simulink model "single_magnet_single_superconductor"  (R2014a)
settings: Solver=ode45  StartTime=0.0  StopTime=sim_time  RelTol=1e-16
values from neighbouring files (symbols this model uses):
  damping = evalin('base', 'damping')    [FP_sandbox.m]
  mu_FC = [mu_FC_x; mu_FC_y; mu_FC_z]    [FP_sandbox.m]
  mu_mag_0 = evalin('base','mu_mag_0')    [FP_sandbox.m]
  r_FC = [pos_FC_x; pos_FC_y; pos_FC_z]    [FP_sandbox.m]
  r_mag_0 = evalin('base', 'r_mag_0')    [FP_sandbox.m]
undefined symbols (not defined in the file or in its folder): Quat_A0
libraries: simulink x1, vrlib x1
settings Model: Creator=user  LastModifiedBy=user

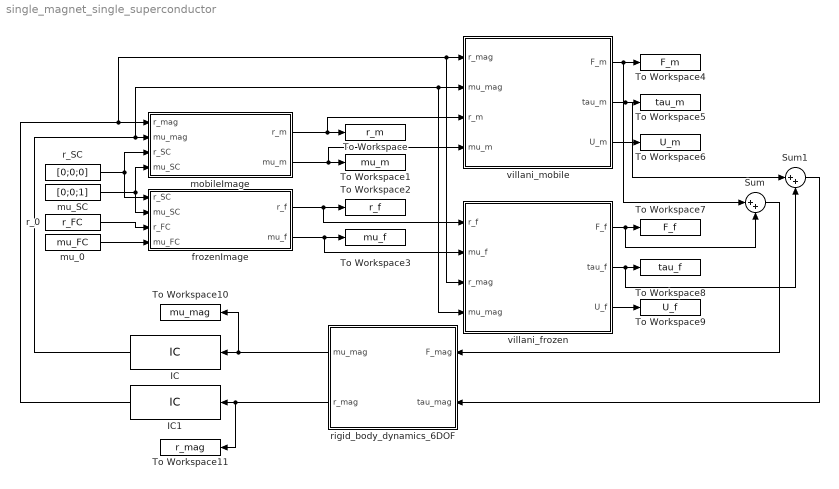
== system single_magnet_single_superconductor ==
  IC : InitialCondition  Value=mu_mag_0
  IC1 : InitialCondition  Value=r_mag_0
  Sum : Sum  Inputs=|++
  Sum1 : Sum  Inputs=|++
  To Workspace : ToWorkspace  VariableName=r_m  SaveFormat=Timeseries  SampleTime=-1
  To Workspace1 : ToWorkspace  VariableName=mu_m  SaveFormat=Timeseries  SampleTime=-1
  To Workspace10 : ToWorkspace  VariableName=mu_mag  SaveFormat=Timeseries  SampleTime=-1
  To Workspace11 : ToWorkspace  VariableName=r_mag  SaveFormat=Timeseries  SampleTime=-1
  To Workspace2 : ToWorkspace  VariableName=r_f  SaveFormat=Timeseries  SampleTime=-1
  To Workspace3 : ToWorkspace  VariableName=mu_f  SaveFormat=Timeseries  SampleTime=-1
  To Workspace4 : ToWorkspace  VariableName=F_m  SaveFormat=Timeseries  SampleTime=-1
  To Workspace5 : ToWorkspace  VariableName=tau_m  SaveFormat=Timeseries  SampleTime=-1
  To Workspace6 : ToWorkspace  VariableName=U_m  SaveFormat=Timeseries  SampleTime=-1
  To Workspace7 : ToWorkspace  VariableName=F_f  SaveFormat=Timeseries  SampleTime=-1
  To Workspace8 : ToWorkspace  VariableName=tau_f  SaveFormat=Timeseries  SampleTime=-1
  To Workspace9 : ToWorkspace  VariableName=U_f  SaveFormat=Timeseries  SampleTime=-1
  frozenImage : MATLAB Function  TreatAsAtomicUnit=on
  mobileImage : MATLAB Function  TreatAsAtomicUnit=on
  mu_0 : Constant  Value=mu_FC
  mu_SC : Constant  Value=[0;0;1]
  r_0 : Constant  Value=r_FC
  r_SC : Constant  Value=[0;0;0]
  "rigid_body_dynamics_6DOF " : Subsystem
  villani_frozen : MATLAB Function  TreatAsAtomicUnit=on
  villani_mobile : MATLAB Function  TreatAsAtomicUnit=on
  wires:
  r_SC/1 -> frozenImage/1(r_SC), mobileImage/3(r_SC)
  mu_SC/1 -> frozenImage/2(mu_SC), mobileImage/4(mu_SC)
  r_0/1 -> frozenImage/3(r_FC)
  mu_0/1 -> frozenImage/4(mu_FC)
  IC/1 -> villani_frozen/4(mu_mag), villani_mobile/2(mu_mag), mobileImage/2(mu_mag)
  IC1/1 -> villani_frozen/3(r_mag), villani_mobile/1(r_mag), mobileImage/1(r_mag)
  mobileImage/1(r_m) -> villani_mobile/3(r_m), To Workspace/1
  mobileImage/2(mu_m) -> villani_mobile/4(mu_m), To Workspace1/1
  frozenImage/1(r_f) -> villani_frozen/1(r_f), To Workspace2/1
  frozenImage/2(mu_f) -> villani_frozen/2(mu_f), To Workspace3/1
  villani_mobile/1(F_m) -> Sum/1, To Workspace4/1
  villani_mobile/2(tau_m) -> Sum1/1, To Workspace5/1
  villani_mobile/3(U_m) -> To Workspace6/1
  villani_frozen/1(F_f) -> Sum/2, To Workspace7/1
  villani_frozen/2(tau_f) -> Sum1/2, To Workspace8/1
  villani_frozen/3(U_f) -> To Workspace9/1
  Sum1/1 -> "rigid_body_dynamics_6DOF "/2(tau_mag)
  Sum/1 -> "rigid_body_dynamics_6DOF "/1(F_mag)
  "rigid_body_dynamics_6DOF "/1(mu_mag) -> To Workspace10/1, IC/1
  "rigid_body_dynamics_6DOF "/2(r_mag) -> To Workspace11/1, IC1/1

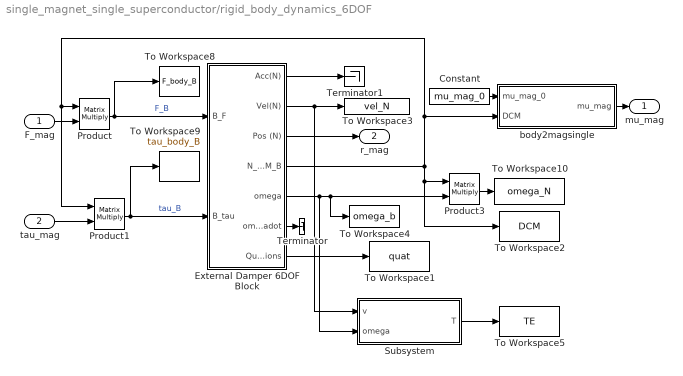
== system single_magnet_single_superconductor/rigid_body_dynamics_6DOF  ==
  F_mag : Inport
  tau_mag : Inport  Port=2
  Constant : Constant  Value=mu_mag_0
  External Damper 6DOF Block : Subsystem  AncestorBlock=OS_Sim_library/External Damper 6DOF block Collision Block
  Product : Product  Multiplication=Matrix(*)
  Product1 : Product  Multiplication=Matrix(*)
  Product3 : Product  Multiplication=Matrix(*)
  Subsystem : Subsystem
  Terminator : Terminator
  Terminator1 : Terminator
  To Workspace1 : ToWorkspace  VariableName=quat  SaveFormat=Timeseries  SampleTime=-1
  To Workspace10 : ToWorkspace  VariableName=omega_N  SaveFormat=Timeseries  SampleTime=-1
  To Workspace2 : ToWorkspace  VariableName=DCM  SaveFormat=Structure With Time  SampleTime=-1
  To Workspace3 : ToWorkspace  VariableName=vel_N  SaveFormat=Timeseries  SampleTime=-1
  To Workspace4 : ToWorkspace  VariableName=omega_b  SaveFormat=Timeseries  SampleTime=-1
  To Workspace5 : ToWorkspace  VariableName=TE  SaveFormat=Timeseries  SampleTime=-1
  To Workspace8 : ToWorkspace  VariableName=F_body_B  SaveFormat=Timeseries  SampleTime=-1
  To Workspace9 : ToWorkspace  VariableName=tau_body_B  SaveFormat=Timeseries  SampleTime=-1
  body2magsingle : MATLAB Function  TreatAsAtomicUnit=on
  mu_mag : Outport
  r_mag : Outport  Port=2
  wires:
  External Damper 6DOF Block/1(Acc(N)) -> Terminator1/1
  External Damper 6DOF Block/6(omegadot) -> Terminator/1
  External Damper 6DOF Block/2(Vel(N)) -> Subsystem/1(v), To Workspace3/1
  body2magsingle/1(mu_mag) -> mu_mag/1
  tau_mag/1 -> Product1/2
  F_mag/1 -> Product/2
  External Damper 6DOF Block/4(N_DCM_B) -> Product1/1, Product/1, body2magsingle/2(DCM), Product3/1, To Workspace2/1
  Product1/1 -> External Damper 6DOF Block/2(B_tau), To Workspace9/1  "tau_B"
  Product/1 -> External Damper 6DOF Block/1(B_F), To Workspace8/1  "F_B"
  External Damper 6DOF Block/3(Pos (N)) -> r_mag/1
  Product3/1 -> To Workspace10/1
  External Damper 6DOF Block/5(omega) -> Product3/2, To Workspace4/1, Subsystem/2(omega)
  External Damper 6DOF Block/7(Quaternions) -> To Workspace1/1
  Subsystem/1(T) -> To Workspace5/1
  Constant/1 -> body2magsingle/1(mu_mag_0)

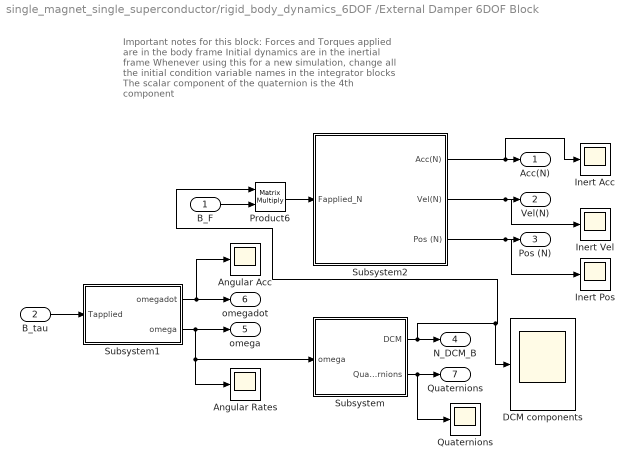
== system single_magnet_single_superconductor/rigid_body_dynamics_6DOF /External Damper 6DOF Block ==
  note: Important notes for this block:
      | Forces and Torques applied are in the body frame
      | Initial dynamics are in the inertial frame
      | Whenever using this for a new simulation, change all the initial condition variable names in the integrator blocks
      | The scalar component of the quaternion is the 4th component
  B_F : Inport
  B_tau : Inport  Port=2
  Angular Acc : Scope
      settings: SaveName=ScopeData30
  Angular Rates : Scope
      settings: SaveName=ScopeData31
  DCM components : Scope
      settings: SaveName=ScopeData34
  Inert Acc : Scope
      settings: SaveName=ScopeData20
  Inert Pos : Scope
      settings: SaveName=ScopeData22
  Inert Vel : Scope
      settings: SaveName=ScopeData21
  Product6 : Product  Multiplication=Matrix(*)  RndMeth=Zero
  "Quaternions " : Scope
      settings: SaveName=ScopeData33
  Subsystem : Subsystem
  Subsystem1 : Subsystem
  Subsystem2 : Subsystem
  Acc(N) : Outport
  Vel(N) : Outport  Port=2  PortDimensions=[3 1]
  Pos (N) : Outport  Port=3
  N_DCM_B : Outport  Port=4
  omega : Outport  Port=5  PortDimensions=[3 1]
  omegadot : Outport  Port=6
  Quaternions : Outport  Port=7
  wires:
  Product6/1 -> Subsystem2/1(Fapplied_N)
  Subsystem/2(Quaternions) -> Quaternions/1, "Quaternions "/1
  Subsystem/1(DCM) -> N_DCM_B/1, Product6/1, DCM components/1
  Subsystem1/1(omegadot) -> omegadot/1, Angular Acc/1
  Subsystem1/2(omega) -> Angular Rates/1, Subsystem/1(omega), omega/1
  B_tau/1 -> Subsystem1/1(Tapplied)
  Subsystem2/1(Acc(N)) -> Inert Acc/1, Acc(N)/1
  Subsystem2/2(Vel(N)) -> Inert Vel/1, Vel(N)/1
  Subsystem2/3(Pos (N)) -> Inert Pos/1, Pos (N)/1
  B_F/1 -> Product6/2

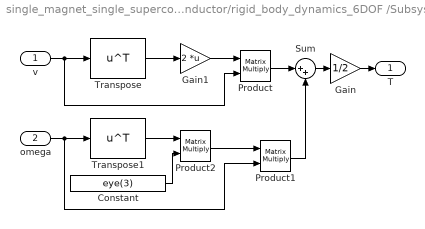
== system single_magnet_single_superconductor/rigid_body_dynamics_6DOF /Subsystem ==
  v : Inport
  omega : Inport  Port=2
  Constant : Constant  Value=eye(3)
  Gain : Gain  Gain=1/2
  Gain1 : Gain  Gain=2  Multiplication=Matrix(K*u)
  Product : Product  Multiplication=Matrix(*)
  Product1 : Product  Multiplication=Matrix(*)
  Product2 : Product  Multiplication=Matrix(*)
  Sum : Sum  Inputs=|++
  Transpose : Math  Operator=transpose  SaturateOnIntegerOverflow=on
  Transpose1 : Math  Operator=transpose  SaturateOnIntegerOverflow=on
  T : Outport  PortDimensions=1
  wires:
  v/1 -> Product/2, Transpose/1
  Transpose/1 -> Gain1/1
  Gain1/1 -> Product/1
  Sum/1 -> Gain/1
  Gain/1 -> T/1
  omega/1 -> Product1/2, Transpose1/1
  Transpose1/1 -> Product2/1
  Product2/1 -> Product1/1
  Product/1 -> Sum/1
  Product1/1 -> Sum/2
  Constant/1 -> Product2/2

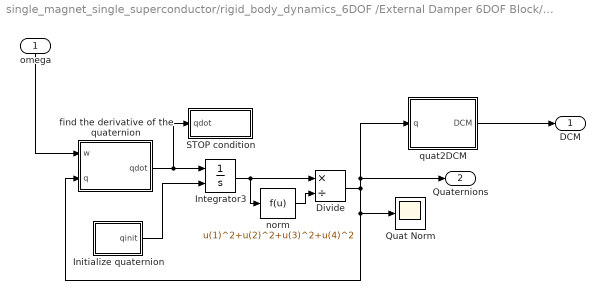
== system single_magnet_single_superconductor/rigid_body_dynamics_6DOF /External Damper 6DOF Block/Subsystem ==
  omega : Inport
  Divide : Product  Inputs=*/
  Initialize quaternion : Subsystem
  Integrator3 : Integrator  InitialConditionSource=external  InitialCondition=Quat_A0
  Quat Norm : Scope
      settings: YMin=-0.1  YMax=1  SaveName=ScopeData32
  STOP condition : Subsystem
  find the derivative of the quaternion : MATLAB Function  TreatAsAtomicUnit=on
  norm : Fcn  Expr=u(1)^2+u(2)^2+u(3)^2+u(4)^2
  quat2DCM : MATLAB Function  TreatAsAtomicUnit=on
  DCM : Outport
  Quaternions : Outport  Port=2
  wires:
  Initialize quaternion/1(qinit) -> Integrator3/2
  quat2DCM/1(DCM) -> DCM/1
  find the derivative of the quaternion/1(qdot) -> STOP condition/1(qdot), Integrator3/1
  Divide/1 -> quat2DCM/1(q), Quaternions/1, find the derivative of the quaternion/2(q), Quat Norm/1
  Integrator3/1 -> Divide/1, norm/1
  omega/1 -> find the derivative of the quaternion/1(w)
  norm/1 -> Divide/2

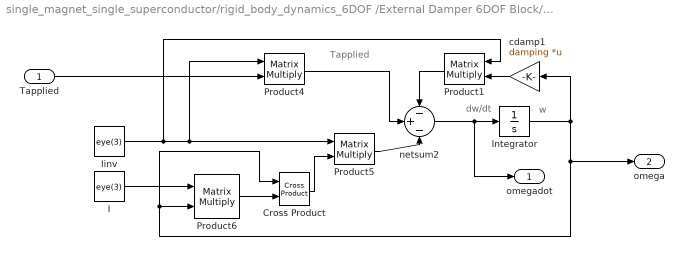
== system single_magnet_single_superconductor/rigid_body_dynamics_6DOF /External Damper 6DOF Block/Subsystem1 ==
  note: dw/dt
  note: w
  note: Tapplied
  Tapplied : Inport
  Cross Product : vrlib/Utilities/Cross Product
  I : Constant  Value=eye(3)  VectorParams1D=off
  Iinv : Constant  Value=eye(3)  VectorParams1D=off
  Integrator : Integrator  InitialCondition=[0 0 0]'
  Product{1,4..6} (4 alike) : Product  Multiplication=Matrix(*)  RndMeth=Zero
  cdamp1 : Gain  Gain=damping  Multiplication=Matrix(K*u)
  netsum2 : Sum  Inputs=-+-  SaturateOnIntegerOverflow=on  InputSameDT=on  OutDataTypeStr=Inherit: Same as first input
  omegadot : Outport
  omega : Outport  Port=2
  wires:
  Cross Product/1 -> Product5/2
  Product4/1 -> netsum2/2
  Product5/1 -> netsum2/3
  Iinv/1 -> Product1/1, Product4/1, Product5/1
  Tapplied/1 -> Product4/2
  Product6/1 -> Cross Product/2
  I/1 -> Product6/1
  netsum2/1 -> Integrator/1, omegadot/1
  Integrator/1 -> omega/1, Cross Product/1, Product6/2, cdamp1/1
  cdamp1/1 -> Product1/2
  Product1/1 -> netsum2/1

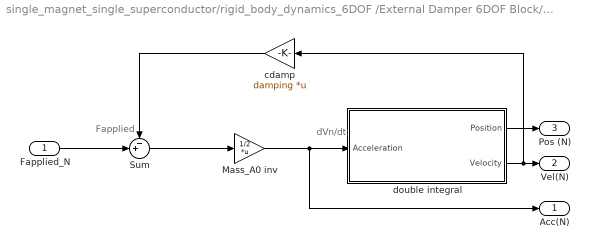
== system single_magnet_single_superconductor/rigid_body_dynamics_6DOF /External Damper 6DOF Block/Subsystem2 ==
  note: dVn/dt
  note: Fapplied
  Fapplied_N : Inport
  Mass_A0 inv : Gain  Gain=1/2  Multiplication=Matrix(K*u)
  Sum : Sum  Inputs=-+|  SaturateOnIntegerOverflow=on
  cdamp : Gain  Gain=damping  Multiplication=Matrix(K*u)
  double integral : Subsystem
  Acc(N) : Outport
  Vel(N) : Outport  Port=2
  Pos (N) : Outport  Port=3
  wires:
  double integral/2(Velocity) -> Vel(N)/1, cdamp/1
  double integral/1(Position) -> Pos (N)/1
  Mass_A0 inv/1 -> double integral/1(Acceleration), Acc(N)/1
  Sum/1 -> Mass_A0 inv/1
  Fapplied_N/1 -> Sum/2
  cdamp/1 -> Sum/1

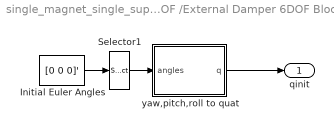
== system single_magnet_single_superconductor/rigid_body_dynamics_6DOF /External Damper 6DOF Block/Subsystem/Initialize quaternion ==
  Initial Euler Angles : Constant  Value=[0 0 0]'
  Selector1 : Selector  InputPortWidth=3  Indices=[3 2 1]
  yaw,pitch,roll to quat : MATLAB Function  TreatAsAtomicUnit=on
  qinit : Outport
  wires:
  yaw,pitch,roll to quat/1(q) -> qinit/1
  Selector1/1 -> yaw,pitch,roll to quat/1(angles)
  Initial Euler Angles/1 -> Selector1/1

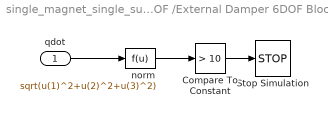
== system single_magnet_single_superconductor/rigid_body_dynamics_6DOF /External Damper 6DOF Block/Subsystem/STOP condition ==
  qdot : Inport
  Compare To Constant : simulink/Logic and Bit Operations/Compare To Constant  relop=>  const=10  OutDataTypeStr=boolean
  Stop Simulation : Stop
  norm : Fcn  Expr=sqrt(u(1)^2+u(2)^2+u(3)^2)
  wires:
  Compare To Constant/1 -> Stop Simulation/1
  norm/1 -> Compare To Constant/1
  qdot/1 -> norm/1

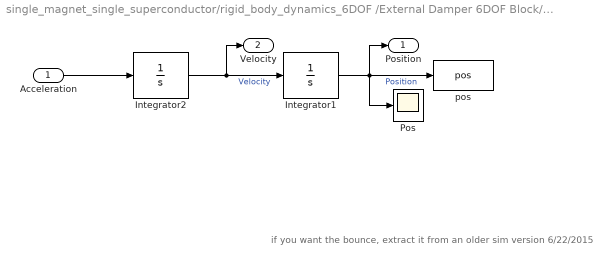
== system single_magnet_single_superconductor/rigid_body_dynamics_6DOF /External Damper 6DOF Block/Subsystem2/double integral ==
  note: if you want the bounce, extract it from an older sim version 6/22/2015
  Acceleration : Inport
  Integrator1 : Integrator  InitialCondition=r_mag_0
  Integrator2 : Integrator  InitialCondition=[0 0 0]'  UpperSaturationLimit=100  LowerSaturationLimit=-100
  Pos : Scope
  pos : ToWorkspace  VariableName=pos  SaveFormat=Timeseries  SampleTime=-1
  Position : Outport
  Velocity : Outport  Port=2
  wires:
  Acceleration/1 -> Integrator2/1
  Integrator2/1 -> Integrator1/1, Velocity/1  "Velocity"
  Integrator1/1 -> pos/1, Position/1, Pos/1  "Position"

== matlab function single_magnet_single_superconductor/frozenImage ==
  data: r_SC input; mu_SC input; r_f output; r_FC input; mu_FC input; mu_f output
function [r_f,mu_f]= frozenImage(r_SC,mu_SC,r_FC,mu_FC)
%#codegen

mu_f=mu_FC;
r_f=r_FC-2*dot((r_FC-r_SC),mu_SC)*mu_SC;

== matlab function single_magnet_single_superconductor/mobileImage ==
  data: r_mag input; mu_mag input; r_SC input; mu_SC input; r_m output; mu_m output
function [r_m,mu_m]= mobileImage(r_mag,mu_mag,r_SC,mu_SC)
%#codegen

mu_m=mu_mag-2*dot(mu_SC,mu_mag)*mu_SC;
r_m=r_mag-2*dot((r_mag-r_SC),mu_SC)*mu_SC;

== matlab function single_magnet_single_superconductor/villani_mobile ==
  data: r_mag input; mu_mag input; r_m input; F_m output; mu_m input; tau_m output; U_m output
function [F_m, tau_m, U_m] = villani_mobile(r_mag,mu_mag,r_m,mu_m)
%#codegen
%all equations taken from Yung/Villani Force and Torque Between Magnetic Dipoles
%test script named Villani_test, passed all test cases in Villani force paper

%the permeability of free space, mu_0
mu_0=4*pi*10^-7; %N/A^2

mu_m_norm=norm(mu_m);
mu_m_hat=mu_m/mu_m_norm;

mu_mag_norm=norm(mu_mag);
mu_mag_hat=mu_mag/mu_mag_norm;

rho=r_mag-r_m;
rho_norm=norm(rho);
rho_hat=rho/rho_norm;

F_m=3*mu_0*mu_m_norm*mu_mag_norm/4/pi/rho_norm^4*...
    (rho_hat*dot(mu_m_hat,mu_mag_hat)+...
    mu_m_hat*dot(rho_hat,mu_mag_hat)+...
    mu_mag_hat*dot(rho_hat,mu_m_hat)-...
    5*rho_hat*dot(rho_hat,mu_m_hat)*dot(rho_hat,mu_mag_hat));
tau_m=mu_0*mu_m_norm*mu_mag_norm/4/pi/rho_norm^3*...
    (3*dot(mu_m_hat,rho_hat)*cross(mu_mag_hat,rho_hat)+...
    cross(mu_m_hat,mu_mag_hat));

B=mu_0/4/pi*(3*dot(mu_m,rho)*rho/rho_norm^5 ...
    -mu_m/rho_norm^3);
U_m=-dot(mu_mag,B)/2;
end

== matlab function single_magnet_single_superconductor/villani_frozen ==
  data: r_f input; mu_f input; r_mag input; mu_mag input; F_f output; tau_f output; U_f output
function [F_f, tau_f, U_f] = villani_frozen(r_f,mu_f,r_mag,mu_mag)
%#codegen
%all equations taken from Yung/Villani Force and Torque Between Magnetic Dipoles
%test script named Villani_test, passed all test cases in Villani force paper

%the permeability of free space, mu_0
mu_0=4*pi*10^-7; %N/A^2

mu_m_norm=norm(mu_f);
mu_m_hat=mu_f/mu_m_norm;

mu_mag_norm=norm(mu_mag);
mu_mag_hat=mu_mag/mu_mag_norm;

rho=r_mag-r_f;
rho_norm=norm(rho);
rho_hat=rho/rho_norm;

F_f=3*mu_0*mu_m_norm*mu_mag_norm/4/pi/rho_norm^4*...
    (rho_hat*dot(mu_m_hat,mu_mag_hat)+...
    mu_m_hat*dot(rho_hat,mu_mag_hat)+...
    mu_mag_hat*dot(rho_hat,mu_m_hat)-...
    5*rho_hat*dot(rho_hat,mu_m_hat)*dot(rho_hat,mu_mag_hat));
tau_f=mu_0*mu_m_norm*mu_mag_norm/4/pi/rho_norm^3*...
    (3*dot(mu_m_hat,rho_hat)*cross(mu_mag_hat,rho_hat)+...
    cross(mu_m_hat,mu_mag_hat));

B=mu_0/4/pi*(3*dot(mu_f,rho)*rho/rho_norm^5 ...
    -mu_f/rho_norm^3);
U_f=-dot(mu_mag,B);
end

== matlab function single_magnet_single_superconductor/rigid_body_dynamics_6DOF /body2magsingle ==
  data: mu_mag_0 input; mu_mag output; DCM input
function mu_mag = body2mag(mu_mag_0,DCM)
%#codegen

mu_mag=DCM*mu_mag_0;

== matlab function single_magnet_single_superconductor/rigid_body_dynamics_6DOF /External Damper 6DOF Block/Subsystem/Initialize quaternion/yaw,pitch,roll to quat ==
  data: q output; angles input
function q = ang2quat(angles)
%#eml
phi=angles(1);
theta=angles(2);
psi=angles(3);
q1=sin(phi/2)*cos(theta/2)*cos(psi/2)-cos(phi/2)*sin(theta/2)*sin(psi/2);
q2=cos(phi/2)*sin(theta/2)*cos(psi/2)+sin(phi/2)*cos(theta/2)*sin(psi/2);
q3=cos(phi/2)*cos(theta/2)*sin(psi/2)-sin(phi/2)*cos(theta/2)*sin(psi/2);
q4=cos(phi/2)*cos(theta/2)*cos(psi/2)+sin(phi/2)*sin(theta/2)*sin(psi/2);
q=[q1 q2 q3 q4]';

== matlab function single_magnet_single_superconductor/rigid_body_dynamics_6DOF /External Damper 6DOF Block/Subsystem/find the derivative of the quaternion ==
  data: w input; q input; qdot output
function qdot = dquat(w,q)
%#eml
qcrs=[q(4) -q(3) q(2)
      q(3) q(4) -q(1)
      -q(2) q(1) q(4)
      -q(1) -q(2) -q(3)];
qdot=1/2*qcrs*w;

== matlab function single_magnet_single_superconductor/rigid_body_dynamics_6DOF /External Damper 6DOF Block/Subsystem/quat2DCM ==
  data: q input; DCM output
function DCM = quat2DCM(q)
%#eml
q1=q(1); q2=q(2); q3=q(3); q4=q(4); 

DCM=(q4^2-[q1 q2 q3]*[q1 q2 q3]')*eye(3)+...
    2*[q1 q2 q3]'*[q1 q2 q3]+...
    2*q4*[0 -q3 q2; q3 0 -q1; -q2 q1 0];
